simulink model "techgium"  (R2024b)
settings: Solver=VariableStepAuto  StartTime=0.0  StopTime=10  RelTol=1e-3
libraries: fl_lib x7, nesl_utility x6, batteryecm_lib x1, ee_lib x1
settings Model: PacingRate=1.100000  Creator=ranki  LastModifiedBy=ranki

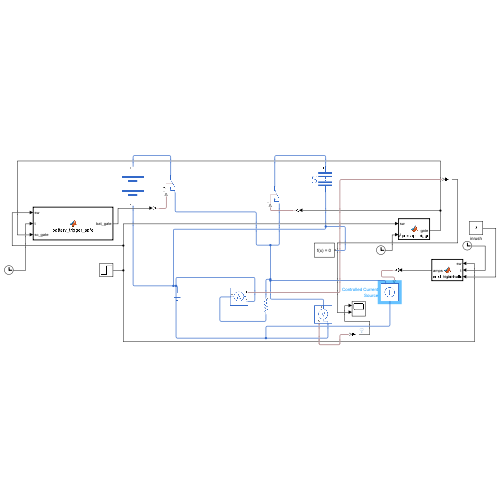
[thumbnail: Simulink's stored preview of the top-level diagram]
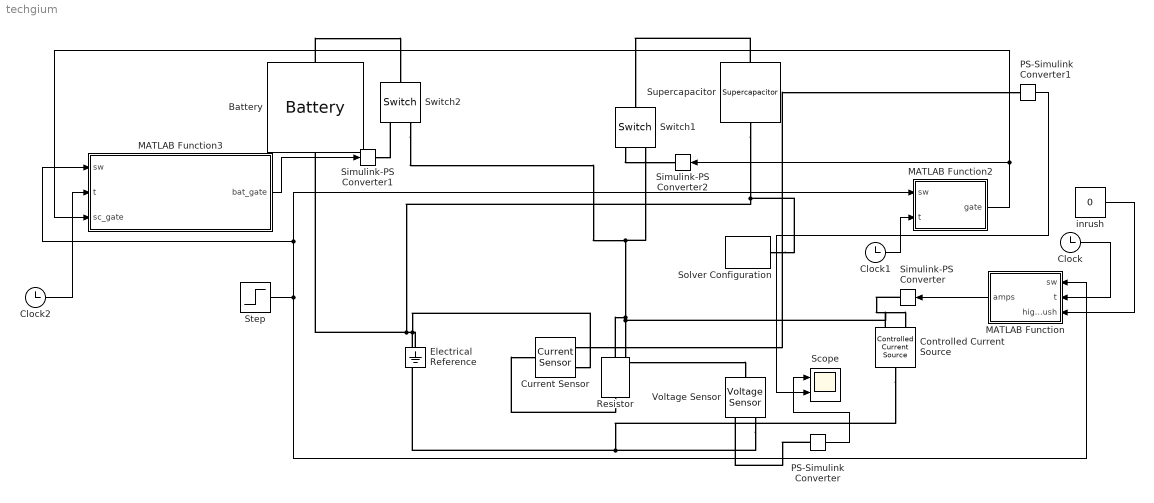
== system techgium ==
  Battery : batteryecm_lib/Battery  Vnom=12 V  prm_dir=simscape.enum.battery.prm_dir.disabled  R1_dis=2 Ohm  R1_ch=2 Ohm  R1=0.01 Ohm  prm_AH=simscape.enum.battery.prm_AH.infinite  AH=50 A*hr  V1=11.5 V  AH1=25 A*hr  prm_R2=simscape.enum.battery.prm_R2.disabled  R2=2000 Ohm  Tmeas=298.15 K  charge_measurement_port=simscape.enum.battery.enable.no  prm_dyn=simscape.enum.battery.prm_dyn.off  Rp1=0.005 Ohm  tau1=30 s  Rp2=0.005 Ohm  tau2=30 s  Rp3=0.005 Ohm  tau3=30 s  Rp4=0.005 Ohm  tau4=30 s  Rp5=0.005 Ohm  tau5=30 s  prm_fade=simscape.enum.battery.prm_fade.disabled  N_fade=100  AH_fade=45 A*hr  R1_fade=2.02 Ohm  R1_ch_fade=2.02 Ohm  V1_fade=10.35 V  prm_age=simscape.enum.battery.prm_age.disabled  prm_age_OCV=simscape.enum.battery.prm_age_OCV.OCV  OCV_age=0.9  SOC_age=60  Tmeas_age=298.15 K  delta_time_age_vec=[0] d  temperature_age_vec=[273] K  OCV_scaling_age=2.2134e6  OCV_offset_age=1.632e6  temp_exp_age=0.515833569 V  t_exp_age=0.75  Vnom_T2=12 V  R1_T2=2.2 Ohm  R1_T2_dis=2.2 Ohm  R1_T2_ch=2.2 Ohm  V1_T2=11.4 V  R2_T2=2200 Ohm  Rp1_T2=0.005 Ohm  tau1_T2=30 s  Rp2_T2=0.005 Ohm  tau2_T2=30 s  Rp3_T2=0.005 Ohm  tau3_T2=30 s  Rp4_T2=0.005 Ohm  tau4_T2=30 s  Rp5_T2=0.005 Ohm  tau5_T2=30 s  Tmeas2=273.15 K  thermal_port=simscape.enum.thermaleffects.omit  thermal_mass=30000 J/K  i_specify=off  i_priority=None  i=0 A  i_nominal_specify=off  i_nominal_value=1  i_nominal_unit=A  v_specify=on  v_priority=None  v=14 V  v_nominal_specify=off  v_nominal_value=1  v_nominal_unit=V  charge_specify=off  charge_priority=High  charge=50 A*hr  charge_nominal_specify=off  charge_nominal_value=1  charge_nominal_unit=A*hr  num_cycles_specify=off  num_cycles_priority=High  num_cycles=0  num_cycles_nominal_specify=off  num_cycles_nominal_value=1  num_cycles_nominal_unit=1  temperature_specify=off  temperature_priority=High  temperature=298.15 K  temperature_nominal_specify=off  temperature_nominal_value=1  temperature_nominal_unit=K
  Clock : Clock
  Clock1 : Clock
  Clock2 : Clock
  Controlled Current Source : fl_lib/Electrical/Electrical Sources/Controlled Current Source
  Current Sensor : fl_lib/Electrical/Electrical Sensors/Current Sensor
  Electrical Reference : fl_lib/Electrical/Electrical Elements/Electrical Reference
  MATLAB Function : MATLAB Function  TreatAsAtomicUnit=on  SystemSampleTime=0.001
  MATLAB Function2 : MATLAB Function  TreatAsAtomicUnit=on  SystemSampleTime=0.001
  MATLAB Function3 : MATLAB Function  TreatAsAtomicUnit=on  SystemSampleTime=0.001
  PS-Simulink Converter : nesl_utility/PS-Simulink Converter  PhysicalDomain=network_engine_domain  SubClassName=ps_output  LeftPortType=input  RightPortType=output  PseudoPeriodic=off  Frequencies=[]  VectorFormat=inherit  Unit=inherit  AffineConversion=off
  PS-Simulink Converter1 : nesl_utility/PS-Simulink Converter  PhysicalDomain=network_engine_domain  SubClassName=ps_output  LeftPortType=input  RightPortType=output  PseudoPeriodic=off  Frequencies=[]  VectorFormat=inherit  Unit=inherit  AffineConversion=off
  Resistor : fl_lib/Electrical/Electrical Elements/Resistor  R=1 Ohm  i_specify=off  i_priority=None  i=0 A  i_nominal_specify=off  i_nominal_value=1  i_nominal_unit=A  v_specify=off  v_priority=None  v=0 V  v_nominal_specify=off  v_nominal_value=1  v_nominal_unit=V
  Scope : Scope  NumInputPorts=2
  Simulink-PS Converter : nesl_utility/Simulink-PS Converter  PhysicalDomain=network_engine_domain  SubClassName=ps_input  LeftPortType=input  RightPortType=output  PseudoPeriodic=off  Frequencies=[]  NoiseDistribution=none  NoiseParameters=[]  Unit=A  AffineConversion=off  FilteringAndDerivatives=provide  SimscapeFilterOrder=1  InputFilterTimeConstant=0.001  UdotUserProvided=0
  Simulink-PS Converter1 : nesl_utility/Simulink-PS Converter  PhysicalDomain=network_engine_domain  SubClassName=ps_input  LeftPortType=input  RightPortType=output  PseudoPeriodic=off  Frequencies=[]  NoiseDistribution=none  NoiseParameters=[]  Unit=1  AffineConversion=off  FilteringAndDerivatives=provide  SimscapeFilterOrder=1  InputFilterTimeConstant=0.001  UdotUserProvided=0
  Simulink-PS Converter2 : nesl_utility/Simulink-PS Converter  PhysicalDomain=network_engine_domain  SubClassName=ps_input  LeftPortType=input  RightPortType=output  PseudoPeriodic=off  Frequencies=[]  NoiseDistribution=none  NoiseParameters=[]  Unit=1  AffineConversion=off  FilteringAndDerivatives=provide  SimscapeFilterOrder=1  InputFilterTimeConstant=0.001  UdotUserProvided=0
  Solver Configuration : nesl_utility/Solver Configuration  PhysicalDomain=network_engine_domain  SubClassName=solver  LeftPortType=input  RightPortType=generic  Tones=[]  Harmonics=[]  SimulateNoise=off  Profile=off  UseLocalSampling=off  EnableSwitchedLinearOptims=on  FrequencyDomain=off  UseCCode=off  RelTol=0.001  AbsTol=0.001  MinStep=1e-09  ToWorkspace=off  RevertToSquareIcSolve=off  NumHomotopyIterations=100  PhasorMode=off  PhasorModeNumHarmonics=1  ConsistencySolver=NEWTON_XTOL_AFTER_FTOL  IndexReductionMethod=DerivativeReplacement  DoDC=off  ResidualTolerance=1e-09  ConsistencyTolSource=GLOBAL  ConsistencyAbsTol=0.001  ConsistencyRelTol=0.001  ConsistencyTolFactor=0.001  UseLocalSolver=off  LocalSolverChoice=NE_BACKWARD_EULER_ADVANCER  ResolveIndetEquations=on  FunctionEvalNumThread=1  LocalSolverSampleTime=0.001  DoFixedCost=off  MaxNonlinIter=3  MaxModeIter=2  ComputeImpulses=off  ImpulseIterations=2  LinearAlgebra=auto  LinearAlgebraNumThread=0  EquationFormulation=NE_TIME_EF  DelaysMemoryBudget=1024  AutomaticFiltering=on  FilteringTimeConstant=0.001  PartitionStorageMethod=AS_NEEDED  PartitionMemoryBudget=1024  PartitionMethod=ROBUST  MultibodyUseLocalSolver=off  MultibodyLocalSolverChoice=ODE1  MultibodyLocalSolverSampleTime=0.001
  Step : Step  Time=3  SampleTime=0
  Supercapacitor : ee_lib/Passive/Supercapacitor  R=[0.02, 0.1, 100] Ohm  C=[100, 10, 20] F  Kv=0.95 F/V  R_discharge=inf Ohm  N_series=5  N_parallel=1  i_specify=off  i_priority=None  i=0 A  i_nominal_specify=off  i_nominal_value=1  i_nominal_unit=A  v_specify=on  v_priority=High  v=12.5 V  v_nominal_specify=off  v_nominal_value=1  v_nominal_unit=V  vc1_specify=off  vc1_priority=High  vc1=0 V  vc1_nominal_specify=off  vc1_nominal_value=1  vc1_nominal_unit=V  vc2_specify=off  vc2_priority=High  vc2=0 V  vc2_nominal_specify=off  vc2_nominal_value=1  vc2_nominal_unit=V  vc3_specify=off  vc3_priority=High  vc3=0 V  vc3_nominal_specify=off  vc3_nominal_value=1  vc3_nominal_unit=V
      settings: InternalSimscapePortConfiguration="{\"Bottom\":[],\"Left\":[{\"id\":\"p\",\"label\":\"+\",\"type\":\"foundation.electrical.electrical\"}],\"Right\":[{\"id\":\"n\",\"label\":\"-\",\"type\":\"foundation.electrical.electrical\"}],\"Top\":[]}"
  Switch1 : fl_lib/Electrical/Electrical Elements/Switch  R_closed=0.01 Ohm  G_open=1e-8 1/Ohm  Threshold=0.5  i_specify=off  i_priority=None  i=0 A  i_nominal_specify=off  i_nominal_value=1  i_nominal_unit=A  v_specify=off  v_priority=None  v=0 V  v_nominal_specify=off  v_nominal_value=1  v_nominal_unit=V
  Switch2 : fl_lib/Electrical/Electrical Elements/Switch  R_closed=0.01 Ohm  G_open=1e-8 1/Ohm  Threshold=0.5  i_specify=off  i_priority=None  i=0 A  i_nominal_specify=off  i_nominal_value=1  i_nominal_unit=A  v_specify=off  v_priority=None  v=0 V  v_nominal_specify=off  v_nominal_value=1  v_nominal_unit=V
  Voltage Sensor : fl_lib/Electrical/Electrical Sensors/Voltage Sensor
  inrush : Constant  Value=0
  wires:
  MATLAB Function2/1(gate) -> Simulink-PS Converter2/1, MATLAB Function3/3(sc_gate)
  Clock1/1 -> MATLAB Function2/2(t)
  Clock2/1 -> MATLAB Function3/2(t)
  Step/1 -> MATLAB Function2/1(sw), MATLAB Function3/1(sw), MATLAB Function/1(sw)
  PS-Simulink Converter/1 -> Scope/1
  MATLAB Function3/1(bat_gate) -> Simulink-PS Converter1/1
  MATLAB Function/1(amps) -> Simulink-PS Converter/1
  Clock/1 -> MATLAB Function/2(t)
  inrush/1 -> MATLAB Function/3(highinrush)
  PS-Simulink Converter1/1 -> Scope/2
  connections:
  Resistor/LConn1 -- Switch2/RConn2 -- Switch1/RConn2 -- Controlled Current Source/RConn2 -- Voltage Sensor/LConn1
  Electrical Reference/LConn1 -- Controlled Current Source/LConn1 -- Voltage Sensor/RConn2 -- Current Sensor/RConn2 -- Solver Configuration/RConn1 -- Supercapacitor/RConn1 -- Battery/RConn1
  PS-Simulink Converter/LConn1 -- Voltage Sensor/RConn1
  Battery/LConn1 -- Switch2/LConn1
  Simulink-PS Converter1/RConn1 -- Switch2/RConn1
  Supercapacitor/LConn1 -- Switch1/LConn1
  Switch1/RConn1 -- Simulink-PS Converter2/RConn1
  Simulink-PS Converter/RConn1 -- Controlled Current Source/RConn1
  Resistor/RConn1 -- Current Sensor/LConn1
  Current Sensor/RConn1 -- PS-Simulink Converter1/LConn1

== matlab function techgium/MATLAB Function2 ==
  settings: updateMethod=DISCRETE
  data: sw input; gate output; t input
function gate = supercap_trigger(sw, t)
% sw = switch input (0 or 1)
% t  = simulation time from Clock block

persistent last_sw;
persistent pulse_start;
persistent pulse_active;

if isempty(last_sw)
    last_sw = 0;
    pulse_active = false;
    pulse_start = 0;
end

% rising edge detection
if sw == 1 && last_sw == 0
    pulse_active = true;
    pulse_start = t;
end

% maintain 2-sec pulse
if pulse_active
    if (t - pulse_start) < 2
        gate = 17;
    else
        gate = 0;
        pulse_active = false;
    end
else
    gate = 0;
end

% update previous switch state
last_sw = sw;
end

== matlab function techgium/MATLAB Function3 ==
  settings: updateMethod=DISCRETE  sampleTime=0.001
  data: sw input; bat_gate output; t input; sc_gate input
function bat_gate = battery_trigger_safe(sw, t, sc_gate)
% bat_gate = battery_trigger_safe(sw, t, sc_gate)
% sw      - switch input (0/1)
% t       - simulation time from Clock block
% sc_gate - current state of supercap gate (0/1)
%
% Output:
% bat_gate becomes 1 only after DELAY seconds from rising edge AND
% after sc_gate has gone low and INTERLOCK seconds passed.

persistent last_sw;
persistent start_time;
persistent active;
persistent last_sc;
persistent sc_off_time;

if isempty(last_sw)
    last_sw = 0;
    start_time = 0;
    active = false;
    last_sc = 0;
    sc_off_time = -1e9; % initialize to a very negative time
end

DELAY = 2.0;        % seconds after rising edge before allowing battery
INTERLOCK = 0.0;    % 10 ms safety interlock after supercap goes LOW

% detect rising edge of the main switch
if sw == 1 && last_sw == 0
    start_time = t;
    active = true;
end

% update supercap-off time when it transitions 1 -> 0
if last_sc == 1 && sc_gate == 0
    sc_off_time = t;
end

% If switch turned off → reset everything
if sw == 0
    active = false;
    bat_gate = 0;
    last_sw = sw;
    last_sc = sc_gate;
    return;
end

% Condition to allow battery gate:
% 1) main delay expired
% 2) supercap gate currently OFF (sc_gate == 0)
% 3) at least INTERLOCK seconds have passed since supercap went OFF
if active && (t - start_time) >= DELAY && sc_gate == 0 && (t - sc_off_time) >= INTERLOCK
    bat_gate = 17;
else
    bat_gate = 0;
end

% update memory states
last_sw = sw;
last_sc = sc_gate;
end

== matlab function techgium/MATLAB Function ==
  data: sw input; amps output; t input; highinrush input
function amps = inrush_controller(sw, t, highinrush)
% This code forces the surge to happen EXACTLY when the system turns on.
persistent active;
persistent start_time;
persistent last_sw;

if isempty(active), active=false; start_time=0; last_sw=0; end

% 1. Detect System Start (Rising Edge of the Switch/Step)
if sw == 1 && last_sw == 0
    active = true;
    start_time = t;
end

% 2. Reset if System turned OFF
if sw == 0
    active = false;
    amps = 0;
    last_sw = sw;
    return;
end

% 3. Apply 50A Surge for the first 0.5 seconds of operation
if active && (t - start_time) <= 0.5
    amps = highinrush; % High Inrush Current
else
    amps = 0;  % Normal Operation
end

last_sw = sw;
end
